simulink model "GCSCustom"  (R2026a)
settings: configuration reference "quad_config" (kept outside this file)
undefined symbols (not defined in the file): landTime, ts_comms
libraries: simulink x7, etargetslib x2
settings Model: DataDictionary=QuadData.sldd  Creator=The MathWorks, Inc.  LastModifiedBy=The MathWorks, Inc.
settings ConfigSetRef: SourceName=quad_config

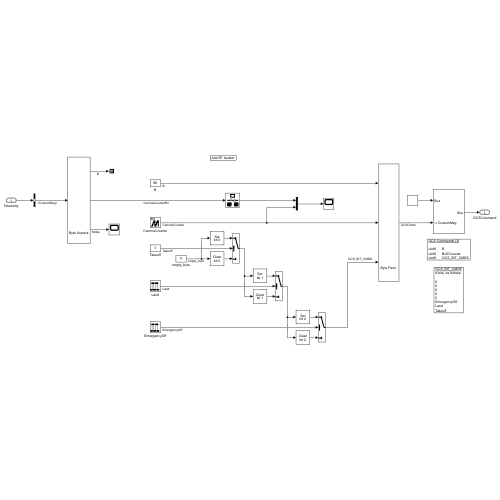
[thumbnail: Simulink's stored preview of the top-level diagram]
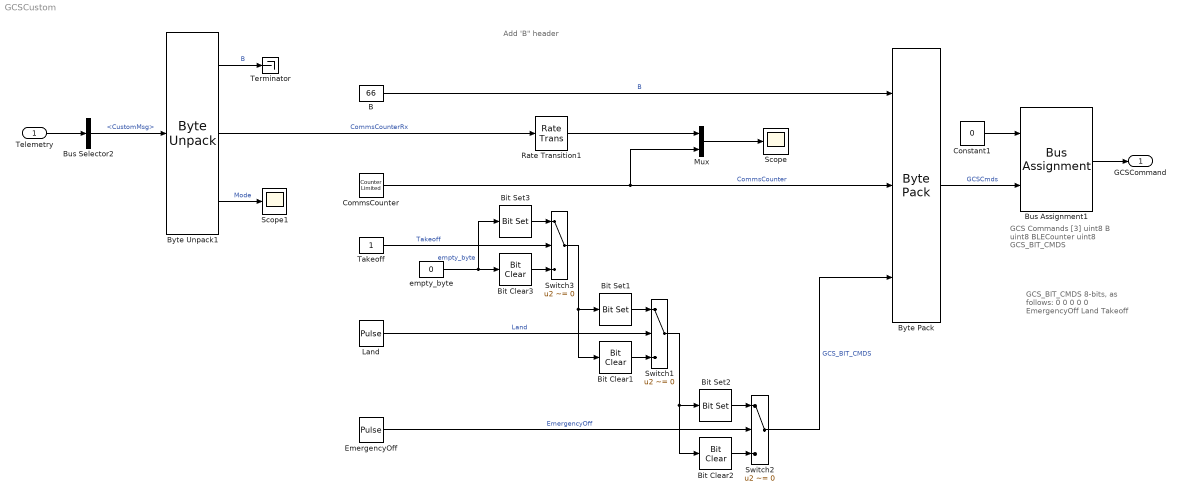
== system GCSCustom ==
  note: Add 'B" header
  note: GCS_BIT_CMDS
      | 8-bits, as follows:
      |
      | 0
      | 0
      | 0
      | 0
      | 0
      | EmergencyOff
      | Land
      | Takeoff
  note: GCS Commands [3]
      |
      | uint8 B
      | uint8 BLECounter
      | uint8 GCS_BIT_CMDS
  Telemetry : Inport  OutDataTypeStr=Bus: Telemetry  BusOutputAsStruct=on
  B : Constant  Value=66  OutDataTypeStr=uint8  SampleTime=-1
  Bit Clear1 : simulink/Logic and Bit Operations/Bit Clear  iBit=1
  Bit Clear2 : simulink/Logic and Bit Operations/Bit Clear  iBit=2
  Bit Clear3 : simulink/Logic and Bit Operations/Bit Clear  iBit=0
  Bit Set1 : simulink/Logic and Bit Operations/Bit Set  iBit=1
  Bit Set2 : simulink/Logic and Bit Operations/Bit Set  iBit=2
  Bit Set3 : simulink/Logic and Bit Operations/Bit Set  iBit=0
  Bus Assignment1 : BusAssignment  AssignedSignals=CustomMsg
  Bus Selector2 : BusSelector  OutputSignals=CustomMsg
  Byte Pack : etargetslib/Byte Pack  datatypes={'uint8' 'uint8' 'uint8'}  byteAlign=1
  Byte Unpack1 : etargetslib/Byte Unpack  dimensions={[1] [1] [1]}  datatypes={'uint8' 'uint8' 'uint8'}  byteAlign=1
  CommsCounter : simulink/Sources/Counter Limited  uplimit=255  tsamp=ts_comms
  Constant1 : Constant  Value=0  OutDataTypeStr=Bus: GCSCmds
  EmergencyOff : DiscretePulseGenerator  Period=50/ts_comms  PulseWidth=0.2/ts_comms  PhaseDelay=30/ts_comms  SampleTime=ts_comms
  Land : DiscretePulseGenerator  Period=50/ts_comms  PulseWidth=0.2/ts_comms  PhaseDelay=landTime/ts_comms  SampleTime=ts_comms
  Mux : Mux  Inputs=2
  Rate Transition1 : RateTransition  Integrity=off  OutPortSampleTime=ts_comms
  Scope : Scope
      settings: ActiveDisplayYMinimum=220.25102  ActiveDisplayYMaximum=262.9252
  Scope1 : Scope
  Switch1 : Switch  Criteria=u2 ~= 0  SaturateOnIntegerOverflow=off  InputSameDT=off
      settings: CopyFcn=AutoSize;  MoveFcn=AutoSize;
  Switch2 : Switch  Criteria=u2 ~= 0  SaturateOnIntegerOverflow=off  InputSameDT=off
      settings: CopyFcn=AutoSize;  MoveFcn=AutoSize;
  Switch3 : Switch  Criteria=u2 ~= 0  SaturateOnIntegerOverflow=off  InputSameDT=off
      settings: CopyFcn=AutoSize;  MoveFcn=AutoSize;
  Takeoff : Constant  OutDataTypeStr=boolean
  Terminator : Terminator
  empty_byte : Constant  Value=0  OutDataTypeStr=uint8
  GCSCommand : Outport  OutDataTypeStr=Bus: GCSCmds
  wires:
  Mux/1 -> Scope/1
  CommsCounter/1 -> Mux/2, Byte Pack/2  "CommsCounter"
  Rate Transition1/1 -> Mux/1
  Switch2/1 -> Byte Pack/3  "GCS_BIT_CMDS"
  Bit Clear3/1 -> Switch3/3
  Bit Set3/1 -> Switch3/1
  Takeoff/1 -> Switch3/2  "Takeoff"
  empty_byte/1 -> Bit Set3/1, Bit Clear3/1  "empty_byte"
  Switch3/1 -> Bit Clear1/1, Bit Set1/1
  Land/1 -> Switch1/2  "Land"
  Bit Set1/1 -> Switch1/1
  Bit Clear1/1 -> Switch1/3
  Bit Clear2/1 -> Switch2/3
  Bit Set2/1 -> Switch2/1
  EmergencyOff/1 -> Switch2/2  "EmergencyOff"
  Switch1/1 -> Bit Clear2/1, Bit Set2/1
  B/1 -> Byte Pack/1  "B"
  Byte Unpack1/1 -> Terminator/1  "B"
  Byte Unpack1/2 -> Rate Transition1/1  "CommsCounterRx"
  Byte Unpack1/3 -> Scope1/1  "Mode"
  Telemetry/1 -> Bus Selector2/1
  Bus Selector2/1 -> Byte Unpack1/1  "<CustomMsg>"
  Constant1/1 -> Bus Assignment1/1
  Bus Assignment1/1 -> GCSCommand/1
  Byte Pack/1 -> Bus Assignment1/2  "GCSCmds"
